simulink model "visotya"  (Simulink 7.3)
settings: Solver=ode45  StartTime=0.0  StopTime=10  RelTol=1e-3
settings Model: Creator=Sainquake  LastModifiedBy=Sainquake Notebook

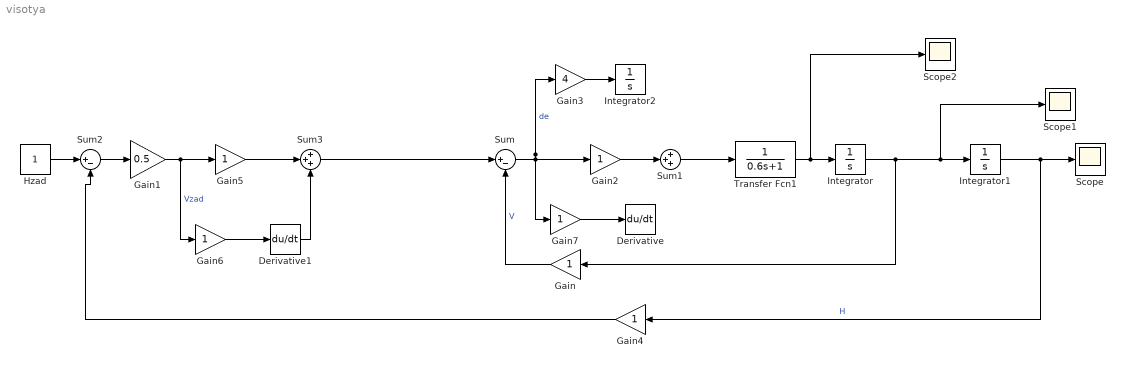
== system visotya ==
  Derivative : Derivative
  Derivative1 : Derivative
  Gain{,2,4..7} (6 alike) : Gain  ParameterDataType=fixdt(1, 16)  ParameterScaling=2^0  OutDataType=fixdt(1, 16)  OutScaling=2^0
  Gain1 : Gain  Gain=0.5  ParameterDataType=fixdt(1, 16)  ParameterScaling=2^0  OutDataType=fixdt(1, 16)  OutScaling=2^0
  Gain3 : Gain  Gain=4  ParameterDataType=fixdt(1, 16)  ParameterScaling=2^0  OutDataType=fixdt(1, 16)  OutScaling=2^0
  Hzad : Constant  OutDataType=fixdt(1, 16)  OutScaling=2^0
  Integrator : Integrator
  Integrator1 : Integrator
  Integrator2 : Integrator
  Scope : Scope
  Scope1 : Scope
  Scope2 : Scope
      settings: SaveName=ScopeData2
  Sum : Sum  Inputs=|+-  OutDataType=fixdt(1, 16)  OutScaling=2^0
  Sum1 : Sum  Inputs=+++  OutDataType=fixdt(1, 16)  OutScaling=2^0
  Sum2 : Sum  Inputs=|+-  OutDataType=fixdt(1, 16)  OutScaling=2^0
  Sum3 : Sum  Inputs=+++  OutDataType=fixdt(1, 16)  OutScaling=2^0
  Transfer Fcn1 : TransferFcn  Numerator=1  Denominator=[0.6 1]
  wires:
  Sum/1 -> Gain2/1, Gain3/1, Gain7/1  "de"
  Transfer Fcn1/1 -> Integrator/1, Scope2/1
  Integrator/1 -> Integrator1/1, Scope1/1, Gain/1
  Integrator1/1 -> Scope/1, Gain4/1  "H"
  Sum1/1 -> Transfer Fcn1/1
  Gain2/1 -> Sum1/2
  Gain3/1 -> Integrator2/1
  Sum2/1 -> Gain1/1
  Hzad/1 -> Sum2/1
  Gain4/1 -> Sum2/2
  Gain/1 -> Sum/2  "V"
  Gain7/1 -> Derivative/1
  Gain5/1 -> Sum3/2
  Gain6/1 -> Derivative1/1
  Gain1/1 -> Gain5/1, Gain6/1  "Vzad"
  Sum3/1 -> Sum/1
  Derivative1/1 -> Sum3/3
